simulink model "simulation_architecture"  (R2021a)
settings: Solver=VariableStepAuto  StartTime=0.0  StopTime=10.0  RelTol=1e-3
InitFcn:
  | global_config
model workspace (MAT data in the model file):
  CG = [0 0 0]
  g = [0 0 -9.81]
  yeet = 3434
libraries: shared6dof x1, vrlib x1
settings Model: Creator=Nabil  LastModifiedBy=Nabil

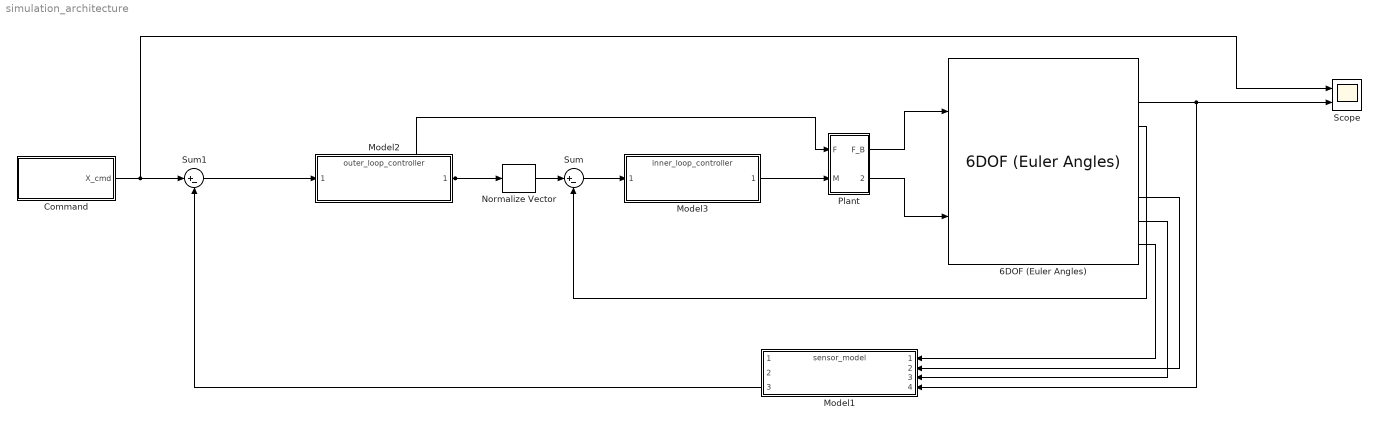
== system simulation_architecture ==
  6DOF (Euler Angles) : shared6dof/6DOF (Euler Angles)  units=Metric (MKS)  mtype=Fixed  rep=Euler Angles  xme_0=[0 0 0]  Vm_0=[0 0 0]  eul_0=[0 0 0]  pm_0=[0 0 0]  mass_0=1.0  mass_e=0.5  mass_f=2.0  inertia=eye(3)  inertia_e=eye(3)  inertia_f=2*eye(3)  k_quat=1.0  vre_flag=on  abi_flag=off  aMode=0  xme_statename=''  Vm_statename=''  eul_statename=''  quat_statename=''  pm_statename=''  mass_statename=''
      settings: SourceProductBaseCode=AE,PW,DR,MT,UV,VE
  Command : Subsystem
  Model1 : ModelReference  ModelNameDialog=sensor_model  SimulationMode=Normal  ModelReferenceVersion=1.2
  Model2 : ModelReference  ModelNameDialog=outer_loop_controller  SimulationMode=Normal  ModelReferenceVersion=1.2
  Model3 : ModelReference  ModelNameDialog=inner_loop_controller  SimulationMode=Normal  ModelReferenceVersion=1.1
  Normalize Vector : vrlib/Utilities/Normalize Vector  maxzero=0
  Plant : Subsystem
  Scope : Scope  NumInputPorts=2
  Sum : Sum  Inputs=|+-
  Sum1 : Sum  Inputs=|+-
  wires:
  6DOF (Euler Angles)/7 -> Model1/3
  6DOF (Euler Angles)/6 -> Model1/2
  6DOF (Euler Angles)/8 -> Model1/1
  6DOF (Euler Angles)/2 -> Scope/2, Model1/4
  6DOF (Euler Angles)/3 -> Sum/2
  Model1/3 -> Sum1/2
  Command/1(X_cmd) -> Scope/1, Sum1/1
  Normalize Vector/1 -> Sum/1
  Model2/1 -> Plant/1(F), Normalize Vector/1
  Sum1/1 -> Model2/1
  Sum/1 -> Model3/1
  Model3/1 -> Plant/2(M)
  Plant/1(F_B) -> 6DOF (Euler Angles)/1
  Plant/2(M_B) -> 6DOF (Euler Angles)/2

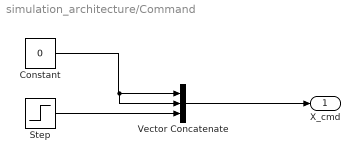
== system simulation_architecture/Command ==
  Constant : Constant  Value=0
  Step : Step  SampleTime=0
  Vector Concatenate : Concatenate  NumInputs=3
  X_cmd : Outport
  wires:
  Vector Concatenate/1 -> X_cmd/1
  Step/1 -> Vector Concatenate/3
  Constant/1 -> Vector Concatenate/2, Vector Concatenate/1

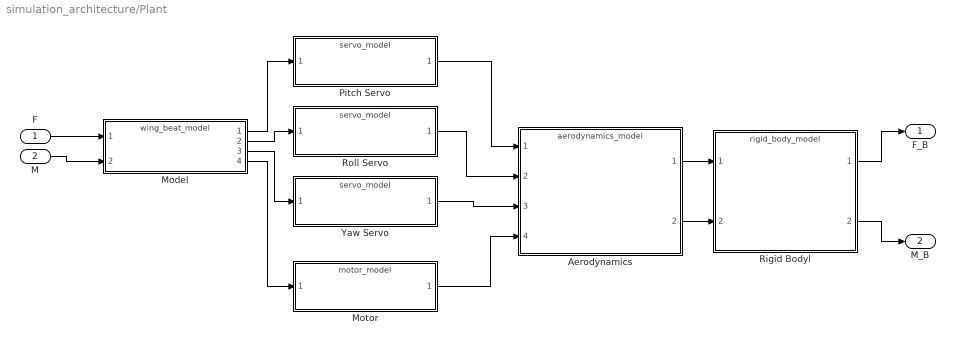
== system simulation_architecture/Plant ==
  F : Inport
  M : Inport  Port=2
  Aerodynamics : ModelReference  ModelNameDialog=aerodynamics_model.slx  SimulationMode=Normal  ModelReferenceVersion=1.4
  Model : ModelReference  ModelNameDialog=wing_beat_model  SimulationMode=Normal  ModelReferenceVersion=1.2
  Motor : ModelReference  ModelNameDialog=motor_model  SimulationMode=Normal  ModelReferenceVersion=1.1
  Pitch Servo : ModelReference  ModelNameDialog=servo_model  SimulationMode=Normal  ModelReferenceVersion=1.1
  Rigid Bodyl : ModelReference  ModelNameDialog=rigid_body_model  SimulationMode=Normal  ModelReferenceVersion=1.2
  Roll Servo : ModelReference  ModelNameDialog=servo_model  SimulationMode=Normal  ModelReferenceVersion=1.1
  Yaw Servo : ModelReference  ModelNameDialog=servo_model  SimulationMode=Normal  ModelReferenceVersion=1.1
  F_B : Outport
  M_B : Outport  Port=2
  wires:
  Aerodynamics/2 -> Rigid Bodyl/2
  Model/2 -> Roll Servo/1
  Model/4 -> Motor/1
  Pitch Servo/1 -> Aerodynamics/1
  Aerodynamics/1 -> Rigid Bodyl/1
  Motor/1 -> Aerodynamics/4
  Roll Servo/1 -> Aerodynamics/2
  Model/3 -> Yaw Servo/1
  Model/1 -> Pitch Servo/1
  Yaw Servo/1 -> Aerodynamics/3
  Rigid Bodyl/1 -> F_B/1
  F/1 -> Model/1
  M/1 -> Model/2
  Rigid Bodyl/2 -> M_B/1
